simulink model "distribution"  (R2015a)
settings: Solver=ode45  StartTime=0  StopTime=1000  RelTol=1e-3
libraries: simulink x1
(part 2 of 2)

== stateflow chart distribution/Element Gamma Recoverable/Chart ==
  state start
    entry: delta_P=dP;
    t_z=0;
    P=P0;
    t0=0;
    i=0;
  state first_sec
    entry:t0=t; i=i+1;dt=t;
    during:P=0;
  state second
    entry:
    tv=t-t0;
    P=P0-dP*i;
    during:tv=t-t0;
    P=P0-dP*i;
  state first
    during: tv=t-t0;
    P=P0-dP*i;
  state third
    entry: t0=t;
    during:P=P0-dP*i;
  (default) -> start
  first -> first_sec : [P<=Pz]
  first_sec -> second : [t-dt>=delta_t]
  start -> first : [t~=0]
  second -> first [order 2] : [P>Pz]
  second -> third [order 1] : [P0==1 && P<=Pz]
  data: dP input; t input; Pz input; delta_P local; t_z local; tv output; P output; i local; t0 local; P0 input; delta_t input; dt local

== stateflow chart distribution/Element Normal Recoverable/Chart ==
  state start
    entry: delta_P=dP;
    t_z=0;
    P=P0;
    t0=0;
    i=0;
  state first_sec
    entry:t0=t; i=i+1;dt=t;
    during:P=0;
  state second
    entry:
    tv=t-t0;
    P=P0-dP*i;
    during:tv=t-t0;
    P=P0-dP*i;
  state first
    during: tv=t-t0;
    P=P0-dP*i;
  state third
    entry: t0=t;
    during:P=P0-dP*i;
  (default) -> start
  first -> first_sec : [P<=Pz]
  first_sec -> second : [t-dt>=delta_t]
  start -> first : [t~=0]
  second -> first [order 2] : [P>Pz]
  second -> third [order 1] : [P0==1 && P<=Pz]
  data: dP input; t input; Pz input; delta_P local; t_z local; tv output; P output; i local; t0 local; P0 input; delta_t input; dt local

== matlab function distribution/Element Gamma Recoverable/Subsystem/G(b) ==
  data: u input; y output
function y = fcn(u)
%#codegen

y = gamma(u);

== stateflow chart distribution/Element Lognormal Recoverable/Chart ==
  state start
    entry: delta_P=dP;
    t_z=0;
    P=P0;
    t0=0;
    i=0;
  state first_sec
    entry:t0=t; i=i+1;dt=t;
    during:P=0;
  state second
    entry:
    tv=t-t0;
    P=P0-dP*i;
    during:tv=t-t0;
    P=P0-dP*i;
  state first
    during: tv=t-t0;
    P=P0-dP*i;
  state third
    entry: t0=t;
    during:P=P0-dP*i;
  (default) -> start
  first -> first_sec : [P<=Pz]
  first_sec -> second : [t-dt>=delta_t]
  start -> first : [t~=0]
  second -> first [order 2] : [P>Pz]
  second -> third [order 1] : [P0==1 && P<=Pz]
  data: dP input; t input; Pz input; delta_P local; t_z local; tv output; P output; i local; t0 local; P0 input; delta_t input; dt local

== matlab function distribution/Element Normal Recoverable/MATLAB Function ==
  data: t input; y output; sigma input; M input
function y = fcn(t,sigma,M)
y=normcdf((t-M)/sigma);

== matlab function distribution/Element Lognormal Recoverable/MATLAB Function ==
  data: t input; y output; sigma input; M input
function y = fcn(t,sigma,M)
y=normcdf((log(t)-M)/sigma);

== stateflow chart distribution/Element Exponental Recoverable /Chart1 ==
  state start
    entry: delta_P=dP;
    t_z=0;
    P=P0;
    t0=0;
    i=0;
  state first_sec
    entry:t0=t; i=i+1;dt=t;
    during:P=0;
  state second
    entry:
    tv=t-t0;
    P=P0-dP*i;
    during:tv=t-t0;
    P=P0-dP*i;
  state first
    during: tv=t-t0;
    P=P0-dP*i;
  state third
    entry: t0=t;
    during:P=P0-dP*i;
  (default) -> start
  first -> first_sec : [P<=Pz]
  first_sec -> second : [t-dt>=delta_t]
  start -> first : [t~=0]
  second -> first [order 2] : [P>Pz]
  second -> third [order 1] : [P0==1 && P<=Pz]
  data: dP input; t input; Pz input; delta_P local; t_z local; tv output; P output; i local; t0 local; P0 input; delta_t input; dt local
